simulink model "PNG_guidanceloop_compensation"  (R2019b)
settings: Solver=FixedStepAuto  StartTime=0.0  StopTime=9.999  FixedStep=0.001  RelTol=1e-3
settings Model: Creator=win10  LastModifiedBy=win10

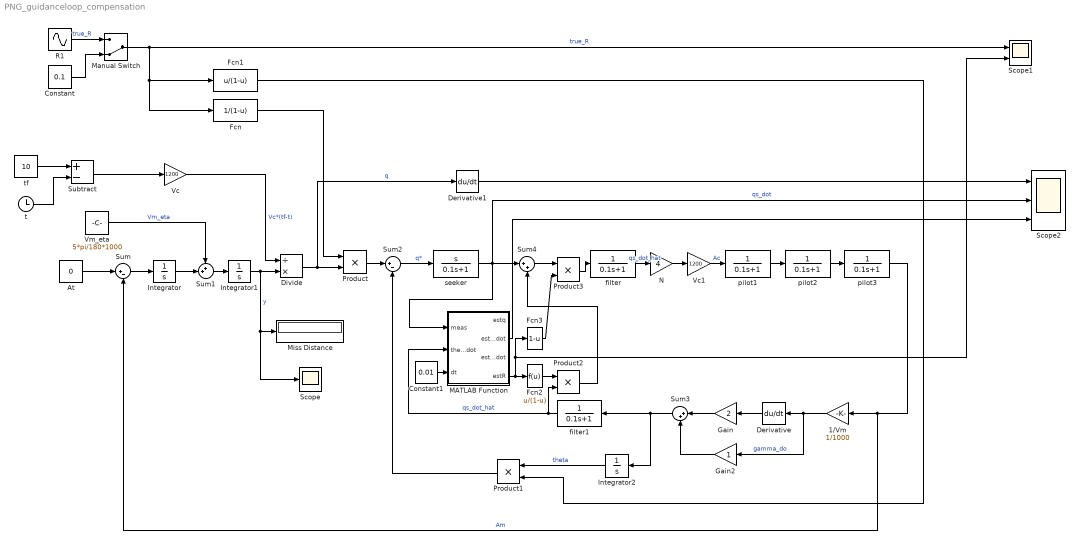
== system PNG_guidanceloop_compensation ==
  1/Vm : Gain  Gain=1/1000
  At : Constant  Value=0
  Constant : Constant  Value=0.1
  Constant1 : Constant  Value=0.01
  Derivative : Derivative
  Derivative1 : Derivative
  Divide : Product  Inputs=/*
  Fcn : Fcn  Expr=1/(1-u)
  Fcn1 : Fcn  Expr=u/(1-u)
  Fcn2 : Fcn  Expr=u/(1-u)
  Fcn3 : Fcn  Expr=1-u
  Gain : Gain  Gain=2
  Gain2 : Gain
  Integrator : Integrator  InitialCondition=120
  Integrator1 : Integrator  InitialCondition=209
  Integrator2 : Integrator  InitialCondition=1*pi/180
  MATLAB Function : MATLAB Function  TreatAsAtomicUnit=on
  Manual Switch : ManualSwitch  CurrentSetting=0
  Miss Distance : Display
  N : Gain  Gain=4
  Product{,1..3} (4 alike) : Product
  R1 : Sin  Amplitude=0.06  Frequency=pi/2  SampleTime=0
  Scope : Scope
  Scope1 : Scope  NumInputPorts=2
  Scope2 : Scope  NumInputPorts=3
  Subtract : Sum  Inputs=+-
  Sum : Sum  Inputs=|+-
  Sum1 : Sum  Inputs=++|
  Sum2 : Sum  Inputs=|+-
  Sum3 : Sum  Inputs=|++
  Sum4 : Sum  Inputs=|++
  Vc : Gain  Gain=1200
  Vc1 : Gain  Gain=1200
  Vm_eta : Constant  Value=5*pi/180*1000
  filter : TransferFcn  Denominator=[0.1 1]
  filter1 : TransferFcn  Denominator=[0.1 1]
  pilot1 : TransferFcn  Denominator=[0.1 1]
  pilot2 : TransferFcn  Denominator=[0.1 1]
  pilot3 : TransferFcn  Denominator=[0.1 1]
  seeker : TransferFcn  Numerator=[1 0]  Denominator=[0.1 1]
  t : Clock
  tf : Constant  Value=10
  wires:
  tf/1 -> Subtract/1
  At/1 -> Sum/1
  Integrator/1 -> Sum1/2
  Sum1/1 -> Integrator1/1
  t/1 -> Subtract/2
  Vm_eta/1 -> Sum1/1  "Vm_eta"
  Subtract/1 -> Vc/1
  Vc/1 -> Divide/1  "Vc*(tf-t)"
  Integrator1/1 -> Miss Distance/1, Scope/1, Divide/2  "y"
  Sum/1 -> Integrator/1
  pilot2/1 -> pilot3/1
  filter/1 -> N/1  "qs_dot_hat"
  Constant/1 -> Manual Switch/2
  Manual Switch/1 -> Scope1/1, Fcn1/1, Fcn/1  "true_R"
  Product/1 -> Sum2/1
  Product1/1 -> Sum2/2
  Sum2/1 -> seeker/1  "q*"
  Vc1/1 -> pilot1/1  "Ac"
  N/1 -> Vc1/1
  R1/1 -> Manual Switch/1  "true_R"
  seeker/1 -> Scope2/2, Sum4/1, MATLAB Function/1(meas)  "qs_dot"
  pilot1/1 -> pilot2/1
  pilot3/1 -> Sum/2, 1/Vm/1  "Am"
  Fcn/1 -> Product/1
  Divide/1 -> Derivative1/1, Product/2  "q"
  Gain/1 -> Sum3/1
  Derivative/1 -> Gain/1
  1/Vm/1 -> Gain2/1, Derivative/1  "gamma_do"
  Gain2/1 -> Sum3/2
  Sum3/1 -> Integrator2/1, filter1/1
  Integrator2/1 -> Product1/1  "theta"
  Fcn1/1 -> Product1/2
  filter1/1 -> Product2/2, MATLAB Function/2(thetaTM_dot)  "qs_dot_hat"
  Constant1/1 -> MATLAB Function/3(dt)
  Fcn2/1 -> Product2/1
  Product2/1 -> Sum4/2
  Sum4/1 -> Product3/1
  Product3/1 -> filter/1
  Fcn3/1 -> Product3/2
  MATLAB Function/4(estR) -> Fcn3/1, Scope1/2, Fcn2/1
  MATLAB Function/2(estq_dot) -> Scope2/3
  Derivative1/1 -> Scope2/1

== matlab function PNG_guidanceloop_compensation/MATLAB Function ==
  settings: updateMethod=DISCRETE  sampleTime=0.01
  data: meas input; estq output; thetaTM_dot input; dt input; estq_dot output; estqst_dot output; estR output
function [estq,estq_dot,estqst_dot,estR] = ExtKalman_Simulink(meas,thetaTM_dot,dt)
% This Embedded MATLAB Function implements an extended Kalman filter used
% for target tracking.
%
% The continuous-time process model is given by
% dx/dt = A*x + B*w

% where, x = [q q_dot qst_dot rou]', q,q_dot is true LOS angle and LOS rate 
% qst_dot is true output of LOS rate from seeker, rou is the radome error
% slope. w = [0 w2 0  w4]'

% Discretize the LTI system model.
%x_k+1 = D*x_k + E*w_k

% and the measurements are given by
% y = qst_dot/(1-rou) - rou/(1-rou)*thetaTM_dot

% Define storage for the variables that need to persist
% between time periods.
Td = 0.1;

persistent P xhat Q R
if isempty(P)
% First time through the code so do some initialization
%  xhat = [0;0;0;0];
%  P = diag([100 100 100 10]);
%  Q = diag([0 1e-5/dt 0 1e-3/dt]);
%  R = diag([0.04*pi*pi/180/180]);
 
  xhat = [0.02;0;0.2;0];
 P = diag([10 10 10 1]);
 Q = diag([0 1e-5 0 1e-3]);
 R = diag([0.04*pi*pi/180/180]);
end


% Calculate the Jacobians for the state equations
% Dynamic state transition matrix in continous-time domain.
A = [0 1 0 0;
     0 0 0 0;
     0 1/Td -1/Td 0;
     0 0 0 0];
  
% noise matrix in continous-time domain.
B = eye(4);
 
% system matrix in discrete-time domain.
% D = expm(A*dt); 
% E = B*dt;

D = [1 dt 0 0;
     0 1 0 0;
     0 dt/Td 1-dt/Td 0;
     0 0 0 1];
E = [dt 0 0 0;
      0 dt 0 0;
      0 0 dt 0;
      0 0 0 dt];
  
    
% % Calculate the Jacobians for the measurement equations
%    q = xhat(1);
%    q_dot = xhat(2);
%    qst_dot = xhat(3);  
%    rou = xhat(4);
%    
% yhat = qst_dot/(1-rou) - rou/(1-rou)*thetaTM_dot;
% 
% H = [0 0 1/(1-rou) (qst_dot-thetaTM_dot)/(1-rou)^2];
%   
% Propogate the state and covariance matrices
xhat = D*xhat;
% xhat = xhat + A*xhat*dt;
P = D*P*D' + E*Q*E';
  
% Calculate the Jacobians for the measurement equations
   q = xhat(1);
   q_dot = xhat(2);
   qst_dot = xhat(3);  
   rou = xhat(4);
   
yhat = qst_dot/(1-rou) - rou/(1-rou)*thetaTM_dot;

H = [0 0 1/(1-rou) (qst_dot-thetaTM_dot)/(1-rou)^2];
    
% Calculate the Kalman gain
K = P*H'/(H*P*H' + R);
% Calculate the measurement residual
resid = meas - yhat;
% Update the state and covariance estimates
xhat = xhat + K*resid;
P = (eye(size(K,1))-K*H)*P;
% Post the results
   estq = xhat(1);
   estq_dot = xhat(2);
   estqst_dot = xhat(3);  
   estR= xhat(4);


% rangeHat = sqrt(xhat(1)^2+xhat(3)^2);
% bearingHat = atan2(xhat(3),xhat(1));
% yu = [thetaM;psiM];
% yhat = MeasurementModel(xhat);
% H = [cos(bearingHat) 0 sin(bearingHat) 0;
%  -sin(bearingHat)/rangeHat 0 cos(bearingHat)/rangeHat 0];
% % Propogate the state and covariance matrices
% xhat = F*xhat;
% P = F*P*F' + Q;
% % Calculate the Kalman gain
% K = P*H'/(H*P*H' + R);
% % Calculate the measurement residual
% resid = meas - yhat;
% % Update the state and covariance estimates
% xhat = xhat + K*resid;
% P = (eye(size(K,1))-K*H)*P;
% % Post the results
% xhatOut = xhat;
% y = u;
